simulink model "Simulink_Lab1.3"  (R2026a)
settings: Solver=FixedStepDiscrete  StopTime=inf  FixedStep=0.001
undefined symbols (not defined in the file or in its folder): Blocking, Non
libraries: simulink x3, amg_usbconverter_n_connect_lib x2
settings Model: Creator=pboon  LastModifiedBy=ACER
settings DebuggingCC: InheritedTsInSrcMsg=none

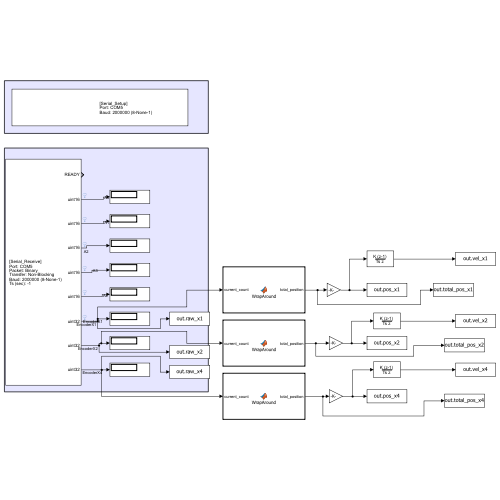
[thumbnail: Simulink's stored preview of the top-level diagram]
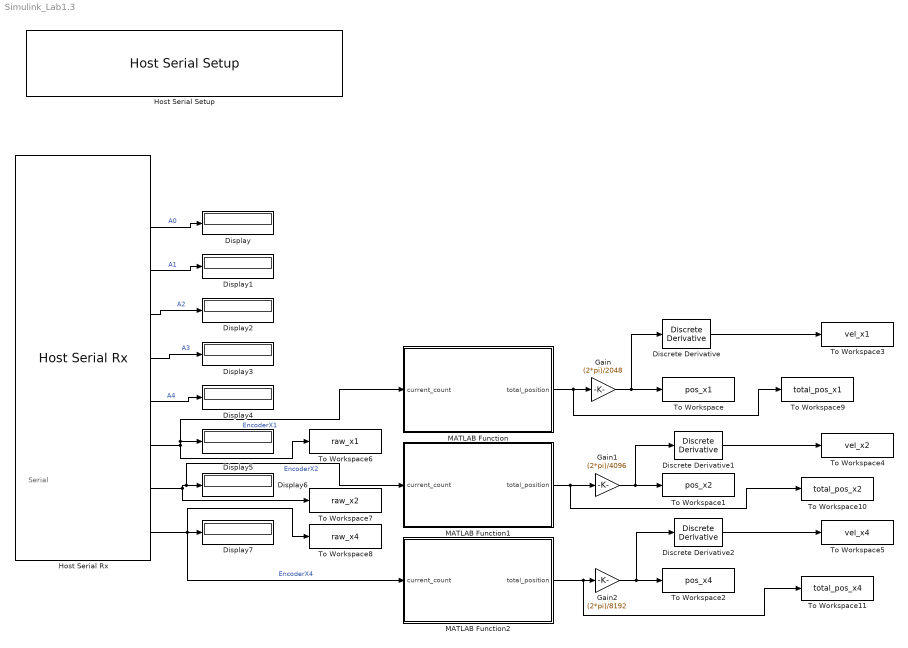
== system Simulink_Lab1.3 ==
  note: Serial
  Discrete Derivative : simulink/Discrete/Discrete Derivative  gainval=1.0  ICPrevScaledInput=0.0  OutMin=[]  OutMax=[]  OutDataType=fixdt(1, 16)  OutScaling=2^-10  DoSatur=off
  Discrete Derivative1 : simulink/Discrete/Discrete Derivative  gainval=1.0  ICPrevScaledInput=0.0  OutMin=[]  OutMax=[]  OutDataType=fixdt(1, 16)  OutScaling=2^-10  DoSatur=off
  Discrete Derivative2 : simulink/Discrete/Discrete Derivative  gainval=1.0  ICPrevScaledInput=0.0  OutMin=[]  OutMax=[]  OutDataType=fixdt(1, 16)  OutScaling=2^-10  DoSatur=off
  Display{,1..7} (8 alike) : Display
  Gain : Gain  Gain=(2*pi)/2048
  Gain1 : Gain  Gain=(2*pi)/4096
  Gain2 : Gain  Gain=(2*pi)/8192
  Host Serial Rx : amg_usbconverter_n_connect_lib/Host Serial Rx  conf=rx  port=COM5  baudrate=2000000  databits=8  parity=None  stopbit=1  flowcontrol=None  transfer=Non-Blocking  timeout=5  packetmode=Binary  enableinitialvalues=off  initialvalues=[]  binheader='25'  binterminator='4E 4E'  porttype_double=0  porttype_single=0  porttype_int8=0  porttype_uint8=0  porttype_int16=0  porttype_uint16=5  porttype_int32=0  porttype_uint32=3  asciiformat='%d,%f'  rx_asciiterminator="CRLF (0x0D 0x0A - \"\\r\\n\")"  tx_asciiterminator="CRLF (0x0D 0x0A - \"\\r\\n\")"  sampletime=0.001  enablecustomportlabel=off  cinputportlabel=0  coutputportlabel=A  portpinstr=0  blockid=HostSerialRx  inputporttype=[]  inputportwidth=[]  inputportlabel={}  outputporttype=[3 5 5 5 5 5 7 7 7]  outputportwidth=[1 1 1 1 1 1 1 1 1]  outputportlabel={'READY','uint16','uint16','uint16','uint16','uint16','uint32','uint32','uint32'}  compat=0  optionstring=[]  autoport='COM5'
  Host Serial Setup : amg_usbconverter_n_connect_lib/Host Serial Setup  conf=setup  port=COM5  baudrate=2000000  databits=8  parity=None  stopbit=1  flowcontrol=None  transfer=Blocking  timeout=2  packetmode=Binary  initialvalues=[]  binheader='7E 7E'  binterminator='03 03'  porttype_double=0  porttype_single=1  porttype_int8=0  porttype_uint8=0  porttype_int16=0  porttype_uint16=0  porttype_int32=0  porttype_uint32=2  asciiformat='%d %u %x'  rx_asciiterminator="CRLF (0x0D 0x0A - \"\\r\\n\")"  tx_asciiterminator="CRLF (0x0D 0x0A - \"\\r\\n\")"  sampletime=-1  enablecustomportlabel=off  cinputportlabel=0  coutputportlabel=A  portpinstr=0  blockid=HostSerialSetup  inputporttype=[]  inputportwidth=[]  inputportlabel={}  outputporttype=[]  outputportwidth=[]  outputportlabel={}  compat=0  optionstring=[]  autoport='COM5'
  MATLAB Function : MATLAB Function  TreatAsAtomicUnit=on
  MATLAB Function1 : MATLAB Function  TreatAsAtomicUnit=on
  MATLAB Function2 : MATLAB Function  TreatAsAtomicUnit=on
  To Workspace : ToWorkspace  VariableName=pos_x1  SaveFormat=Timeseries  SampleTime=-1
  To Workspace1 : ToWorkspace  VariableName=pos_x2  SaveFormat=Timeseries  SampleTime=-1
  To Workspace10 : ToWorkspace  VariableName=total_pos_x2  SaveFormat=Timeseries  SampleTime=-1
  To Workspace11 : ToWorkspace  VariableName=total_pos_x4  SaveFormat=Timeseries  SampleTime=-1
  To Workspace2 : ToWorkspace  VariableName=pos_x4  SaveFormat=Timeseries  SampleTime=-1
  To Workspace3 : ToWorkspace  VariableName=vel_x1  SaveFormat=Timeseries  SampleTime=-1
  To Workspace4 : ToWorkspace  VariableName=vel_x2  SaveFormat=Timeseries  SampleTime=-1
  To Workspace5 : ToWorkspace  VariableName=vel_x4  SaveFormat=Timeseries  SampleTime=-1
  To Workspace6 : ToWorkspace  VariableName=raw_x1  SaveFormat=Timeseries  SampleTime=-1
  To Workspace7 : ToWorkspace  VariableName=raw_x2  SaveFormat=Timeseries  SampleTime=-1
  To Workspace8 : ToWorkspace  VariableName=raw_x4  SaveFormat=Timeseries  SampleTime=-1
  To Workspace9 : ToWorkspace  VariableName=total_pos_x1  SaveFormat=Timeseries  SampleTime=-1
  wires:
  Host Serial Rx/2 -> Display/1  "A0"
  Host Serial Rx/3 -> Display1/1  "A1"
  Host Serial Rx/4 -> Display2/1  "A2"
  Host Serial Rx/5 -> Display3/1  "A3"
  Host Serial Rx/6 -> Display4/1  "A4"
  Host Serial Rx/7 -> To Workspace6/1, MATLAB Function/1(current_count), Display5/1  "EncoderX1"
  Host Serial Rx/8 -> To Workspace7/1, MATLAB Function1/1(current_count), Display6/1  "EncoderX2"
  Host Serial Rx/9 -> To Workspace8/1, MATLAB Function2/1(current_count), Display7/1  "EncoderX4"
  MATLAB Function/1(total_position) -> To Workspace9/1, Gain/1
  MATLAB Function1/1(total_position) -> To Workspace10/1, Gain1/1
  MATLAB Function2/1(total_position) -> To Workspace11/1, Gain2/1
  Gain/1 -> Discrete Derivative/1, To Workspace/1
  Gain1/1 -> Discrete Derivative1/1, To Workspace1/1
  Gain2/1 -> Discrete Derivative2/1, To Workspace2/1
  Discrete Derivative/1 -> To Workspace3/1
  Discrete Derivative1/1 -> To Workspace4/1
  Discrete Derivative2/1 -> To Workspace5/1

== matlab function Simulink_Lab1.3/MATLAB Function ==
  data: current_count input; total_position output
function total_position = WrapAround(current_count)
    
    % 1. แปลงค่า input ให้เป็น double
    current_count = double(current_count);
    
    % *** แก้ตรงนี้: เปลี่ยนเป็นค่าสูงสุดของ 16-bit Timer ***
    MAX_COUNT = 65535; 
    
    % ตั้งค่า Threshold ไว้ประมาณครึ่งหนึ่ง (ใช้ 30000 ได้เหมือนเดิม)
    THRESHOLD = 30000; 
    
    persistent prev_count;
    persistent accumulated_pos;
    
    if isempty(prev_count)
        prev_count = current_count;
        accumulated_pos = 0;
    end
    
    delta = current_count - prev_count;
    
    if delta < -THRESHOLD
        delta = delta + (MAX_COUNT + 1); 
        
    elseif delta > THRESHOLD
        delta = delta - (MAX_COUNT + 1); 
    end
    
    accumulated_pos = accumulated_pos + delta;
    prev_count = current_count;
    total_position = accumulated_pos;
end

== matlab function Simulink_Lab1.3/MATLAB Function2 ==
  data: current_count input; total_position output
function total_position = WrapAround(current_count)
    
    % 1. แปลงค่า input ให้เป็น double
    current_count = double(current_count);
    
    % *** แก้ตรงนี้: เปลี่ยนเป็นค่าสูงสุดของ 16-bit Timer ***
    MAX_COUNT = 65535; 
    
    % ตั้งค่า Threshold ไว้ประมาณครึ่งหนึ่ง (ใช้ 30000 ได้เหมือนเดิม)
    THRESHOLD = 30000; 
    
    persistent prev_count;
    persistent accumulated_pos;
    
    if isempty(prev_count)
        prev_count = current_count;
        accumulated_pos = 0;
    end
    
    delta = current_count - prev_count;
    
    if delta < -THRESHOLD
        delta = delta + (MAX_COUNT + 1); 
        
    elseif delta > THRESHOLD
        delta = delta - (MAX_COUNT + 1); 
    end
    
    accumulated_pos = accumulated_pos + delta;
    prev_count = current_count;
    total_position = accumulated_pos;
end

== matlab function Simulink_Lab1.3/MATLAB Function1 ==
  data: current_count input; total_position output
function total_position = WrapAround(current_count)
    
    % 1. แปลงค่า input ให้เป็น double
    current_count = double(current_count);
    
    % *** แก้ตรงนี้: เปลี่ยนเป็นค่าสูงสุดของ 16-bit Timer ***
    MAX_COUNT = 65535; 
    
    % ตั้งค่า Threshold ไว้ประมาณครึ่งหนึ่ง (ใช้ 30000 ได้เหมือนเดิม)
    THRESHOLD = 30000; 
    
    persistent prev_count;
    persistent accumulated_pos;
    
    if isempty(prev_count)
        prev_count = current_count;
        accumulated_pos = 0;
    end
    
    delta = current_count - prev_count;
    
    if delta < -THRESHOLD
        delta = delta + (MAX_COUNT + 1); 
        
    elseif delta > THRESHOLD
        delta = delta - (MAX_COUNT + 1); 
    end
    
    accumulated_pos = accumulated_pos + delta;
    prev_count = current_count;
    total_position = accumulated_pos;
end
